simulink model "test7"  (R2015a)
settings: Solver=ode45  StartTime=0.0  StopTime=44  RelTol=1e-3
InitFcn:
  | %% DSPBuilder Start
  | alt_dspbuilder_update_model(bdroot)
  | %% DSPBuilder End
libraries: allblocks_alteradspbuilder2 x24
settings Model: Creator=ASUS  LastModifiedBy=ASUS

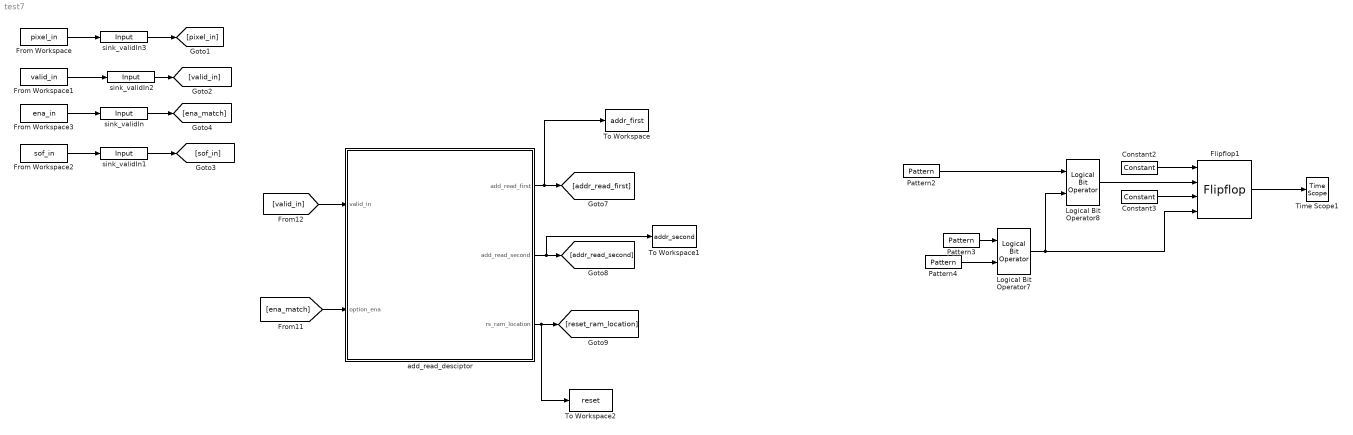
== system test7 ==
  Constant2 : allblocks_alteradspbuilder2/Constant  mask_cst=1  BusType=Unsigned Integer  bwl=1  bwr=0  roundMode=Truncate  satMode=Wrap  SpecifyClock=off  allowFloatingPointOverride=on  logOutputs=off  logFile=C:\Users\ASUS\Desktop\sift_fpga\Octave_2\tb_test7\test7_Constant2.fixedpointlog
  Constant3 : allblocks_alteradspbuilder2/Constant  mask_cst=1  BusType=Unsigned Integer  bwl=1  bwr=0  roundMode=Truncate  satMode=Wrap  SpecifyClock=off  allowFloatingPointOverride=on  logOutputs=off  logFile=C:\Users\ASUS\Desktop\sift_fpga\Octave_2\tb_test7\test7_Constant3.fixedpointlog
  Flipflop1 : allblocks_alteradspbuilder2/Flipflop  mode=DFFE  BusType=Single Bit  bwl=10  bwr=2  pipeline_display=1
  From Workspace : FromWorkspace  VariableName=pixel_in  SampleTime=0
  From Workspace1 : FromWorkspace  VariableName=valid_in  SampleTime=0
  From Workspace2 : FromWorkspace  VariableName=sof_in  SampleTime=0
  From Workspace3 : FromWorkspace  VariableName=ena_in  SampleTime=0
  Logical Bit Operator7 : allblocks_alteradspbuilder2/Logical Bit Operator  LogicalOperator=AND  user_inputs=2  pipeline_display=0
  Logical Bit Operator8 : allblocks_alteradspbuilder2/Logical Bit Operator  LogicalOperator=AND  user_inputs=2  pipeline_display=0
  Pattern2 : allblocks_alteradspbuilder2/Pattern  Sequence=000100010001000100010001000100010001  SpecifyClock=off  use_ena=off  use_sclr=off
  Pattern3 : allblocks_alteradspbuilder2/Pattern  Sequence=011111111111111111111111100000  SpecifyClock=off  use_ena=off  use_sclr=off
  Pattern4 : allblocks_alteradspbuilder2/Pattern  Sequence=11111111111111111111111111111111111111111111  SpecifyClock=off  use_ena=off  use_sclr=off
  Time Scope1 : TimeScope  DefaultConfigurationName=spbscopes.TimeScopeBlockCfg
  To Workspace : ToWorkspace  VariableName=addr_first  SaveFormat=Timeseries  SampleTime=-1
  To Workspace1 : ToWorkspace  VariableName=addr_second  SaveFormat=Timeseries  SampleTime=-1
  To Workspace2 : ToWorkspace  VariableName=reset  SaveFormat=Timeseries  SampleTime=-1
  add_read_desciptor : Subsystem
  sink_validIn : allblocks_alteradspbuilder2/Input  iofile=C:\Users\ASUS\Desktop\sift_fpga\Octave_2\tb_test7\test7_sink%5FvalidIn.salt  BusType=Single Bit  bwl=8  bwr=0  SpecifyClock=off  PORTTYPE=Input  externalType=Inferred  allowFloatingPointOverride=on  logOutputs=off
  sink_validIn1 : allblocks_alteradspbuilder2/Input  iofile=C:\Users\ASUS\Desktop\sift_fpga\Octave_2\tb_test7\test7_sink%5FvalidIn1.salt  BusType=Single Bit  bwl=8  bwr=0  SpecifyClock=off  PORTTYPE=Input  externalType=Inferred  allowFloatingPointOverride=on  logOutputs=off
  sink_validIn2 : allblocks_alteradspbuilder2/Input  iofile=C:\Users\ASUS\Desktop\sift_fpga\Octave_2\tb_test7\test7_sink%5FvalidIn2.salt  BusType=Single Bit  bwl=8  bwr=0  SpecifyClock=off  PORTTYPE=Input  externalType=Inferred  allowFloatingPointOverride=on  logOutputs=off
  sink_validIn3 : allblocks_alteradspbuilder2/Input  iofile=C:\Users\ASUS\Desktop\sift_fpga\Octave_2\tb_test7\test7_sink%5FvalidIn3.salt  BusType=Unsigned Integer  bwl=8  bwr=0  SpecifyClock=off  PORTTYPE=Input  externalType=Inferred  allowFloatingPointOverride=on  logOutputs=off
  wires:
  [valid_in] -> add_read_desciptor/1(valid_in)
  [ena_match] -> add_read_desciptor/2(option_ena)
  add_read_desciptor/1(add_read_first) -> To Workspace/1, [addr_read_first]
  add_read_desciptor/2(add_read_second) -> To Workspace1/1, [addr_read_second]
  add_read_desciptor/3(rs_ram_location) -> To Workspace2/1, [reset_ram_location]
  From Workspace/1 -> sink_validIn3/1
  From Workspace3/1 -> sink_validIn/1
  From Workspace1/1 -> sink_validIn2/1
  sink_validIn/1 -> [ena_match]
  sink_validIn2/1 -> [valid_in]
  sink_validIn3/1 -> [pixel_in]
  From Workspace2/1 -> sink_validIn1/1
  sink_validIn1/1 -> [sof_in]
  Constant2/1 -> Flipflop1/1
  Logical Bit Operator8/1 -> Flipflop1/2
  Constant3/1 -> Flipflop1/3
  Logical Bit Operator7/1 -> Logical Bit Operator8/2, Flipflop1/4
  Flipflop1/1 -> Time Scope1/1
  Pattern4/1 -> Logical Bit Operator7/2
  Pattern3/1 -> Logical Bit Operator7/1
  Pattern2/1 -> Logical Bit Operator8/1

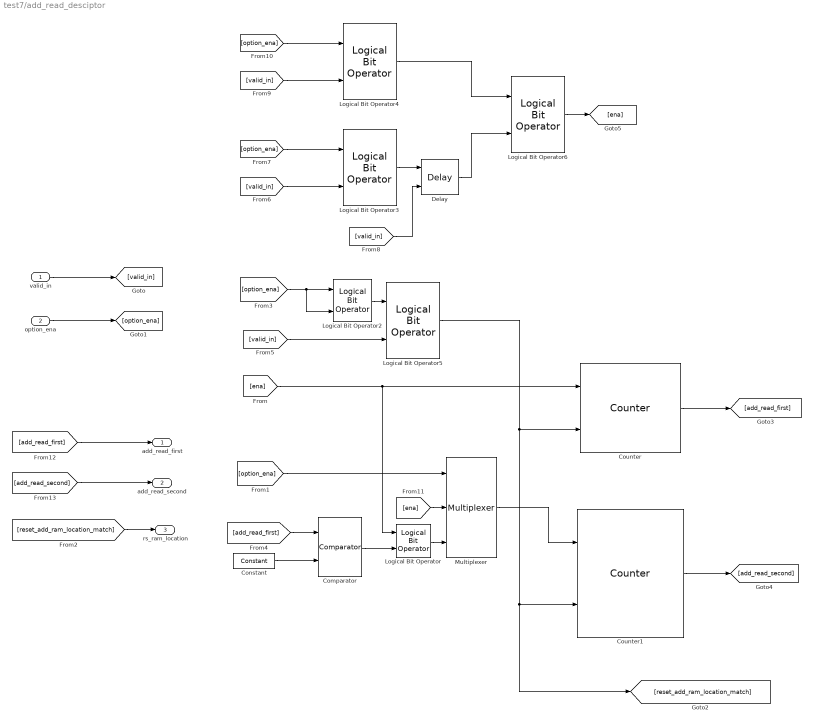
== system test7/add_read_desciptor ==
  valid_in : Inport
  option_ena : Inport  Port=2
  Comparator : allblocks_alteradspbuilder2/Comparator  direction=a == b  pipeline_display=0  allowFloatingPointOverride=on  logOutputs=off  logFile=C:\Users\ASUS\Desktop\sift_fpga\Octave_2\tb_test7\test7_add%5Fread%5Fdesciptor_Comparator.fixedpointlog
  Constant : allblocks_alteradspbuilder2/Constant  mask_cst=999  BusType=Unsigned Integer  bwl=10  bwr=0  roundMode=Truncate  satMode=Wrap  SpecifyClock=off  allowFloatingPointOverride=on  logOutputs=off  logFile=C:\Users\ASUS\Desktop\sift_fpga\Octave_2\tb_test7\test7_add%5Fread%5Fdesciptor_Constant.fixedpointlog
  Counter : allblocks_alteradspbuilder2/Counter  BusType=Unsigned Integer  bwl=10  bwr=0  use_modulo=on  modulo=1000  SpecifyClock=off  direction=Increment  use_sload=off  use_sset=off  svalue=1  use_clk_ena=off  use_ena=on  use_sclr=on  pipeline_display=1
  Counter1 : allblocks_alteradspbuilder2/Counter  BusType=Unsigned Integer  bwl=10  bwr=0  use_modulo=on  modulo=1000  SpecifyClock=off  direction=Increment  use_sload=off  use_sset=off  svalue=0  use_clk_ena=off  use_ena=on  use_sclr=on  pipeline_display=1
  Delay : allblocks_alteradspbuilder2/Delay  pipeline=1  pipeline_display=1  ClockPhase=1  use_ena=on  use_sclr=off  allowFloatingPointOverride=on  logOutputs=off  logFile=C:\Users\ASUS\Desktop\sift_fpga\Octave_2\tb_test7\test7_add%5Fread%5Fdesciptor_Delay.fixedpointlog  use_init=off  reset_value=1
  Logical Bit Operator{,3..5} (4 alike) : allblocks_alteradspbuilder2/Logical Bit Operator  LogicalOperator=AND  user_inputs=2  pipeline_display=0
  Logical Bit Operator2 : allblocks_alteradspbuilder2/Logical Bit Operator  LogicalOperator=NAND  user_inputs=2  pipeline_display=0
  Logical Bit Operator6 : allblocks_alteradspbuilder2/Logical Bit Operator  LogicalOperator=OR  user_inputs=2  pipeline_display=0
  Multiplexer : allblocks_alteradspbuilder2/Multiplexer  numInputs=2  pipeline=0  oneHot=off  pipeline_display=0  use_ena=off  use_aclr=off  allowFloatingPointOverride=on  logOutputs=off  logFile=C:\Users\ASUS\Desktop\sift_fpga\Octave_2\tb_test7\test7_add%5Fread%5Fdesciptor_Multiplexer.fixedpointlog
  add_read_first : Outport
  add_read_second : Outport  Port=2
  rs_ram_location : Outport  Port=3
  wires:
  Logical Bit Operator/1 -> Multiplexer/3
  [add_read_first] -> Comparator/1
  option_ena/1 -> [option_ena]
  Constant/1 -> Comparator/2
  Comparator/1 -> Logical Bit Operator/2
  valid_in/1 -> [valid_in]
  Counter1/1 -> [add_read_second]
  Counter/1 -> [add_read_first]
  [add_read_second] -> add_read_second/1
  [add_read_first] -> add_read_first/1
  [reset_add_ram_location_match] -> rs_ram_location/1
  Logical Bit Operator5/1 -> [reset_add_ram_location_match], Counter1/2, Counter/2
  [option_ena] -> Logical Bit Operator2/2, Logical Bit Operator2/1
  Logical Bit Operator2/1 -> Logical Bit Operator5/1
  [valid_in] -> Logical Bit Operator5/2
  [option_ena] -> Logical Bit Operator3/1
  [valid_in] -> Logical Bit Operator3/2
  Logical Bit Operator3/1 -> Delay/1
  [valid_in] -> Delay/2
  Logical Bit Operator4/1 -> Logical Bit Operator6/1
  [option_ena] -> Logical Bit Operator4/1
  [valid_in] -> Logical Bit Operator4/2
  Delay/1 -> Logical Bit Operator6/2
  Logical Bit Operator6/1 -> [ena]
  [ena] -> Counter/1, Logical Bit Operator/1
  Multiplexer/1 -> Counter1/1
  [option_ena] -> Multiplexer/1
  [ena] -> Multiplexer/2
